simulink model "winter_simulink_with_PC_sim4"  (R2022a)
settings: Solver=VariableStepAuto  StartTime=0  StopTime=stop_time  FixedStep=simulation.time_step_H
undefined symbols (not defined in the file or in its folder): blade, Gc, gearbox, generator, I_eq, lambda_vector, lookup_cP, omega_R, omega_rated, pitch_range, pitch_vector, rho, Riq, rotor, simulation, wind, Yiq
settings Model: Creator=Niccolò  LastModifiedBy=Niccolò

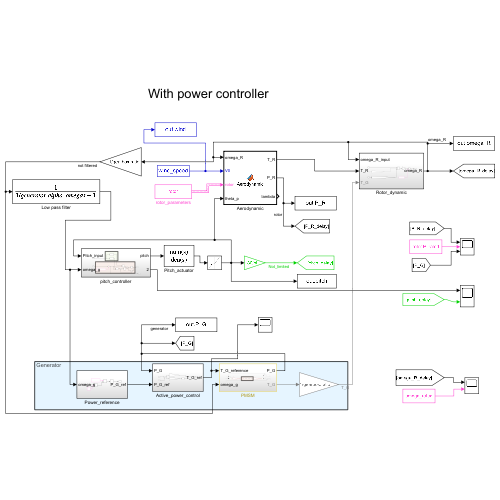
[thumbnail: Simulink's stored preview of the top-level diagram]
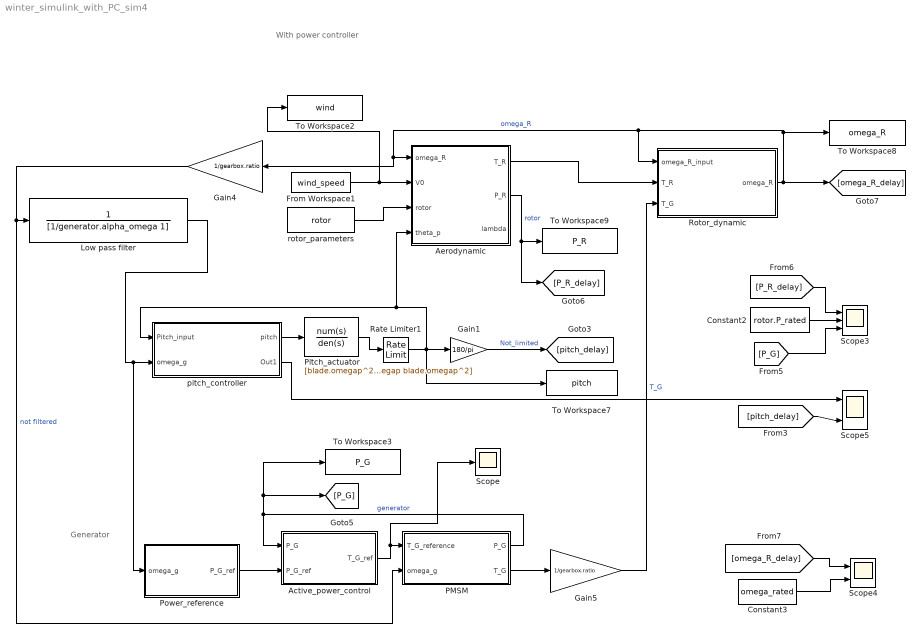
== system winter_simulink_with_PC_sim4 ==
  note: Generator
  note: With power controller
  Active_power_control : Subsystem
  Aerodynamic : MATLAB Function  TreatAsAtomicUnit=on
  Constant2 : Constant  Value=rotor.P_rated
  Constant3 : Constant  Value=omega_rated
  From Workspace1 : FromWorkspace  VariableName=wind_speed  SampleTime=1/wind.sample_f
  Gain1 : Gain  Gain=180/pi  SampleTime=simulation.time_step_H
  Gain4 : Gain  Gain=1/gearbox.ratio
  Gain5 : Gain  Gain=1/gearbox.ratio
  Low pass filter : TransferFcn  Denominator=[1/generator.alpha_omega 1]
  PMSM : Subsystem
  Pitch_actuator : TransferFcn  Numerator=[blade.omegap^2]  Denominator=[1 2*blade.zetap*blade.omegap blade.omegap^2]
  Power_reference : Subsystem
  Rate Limiter1 : RateLimiter  RisingSlewLimit=blade.pitch_rate  FallingSlewLimit=-blade.pitch_rate  SampleTimeMode=inherited
  Rotor_dynamic : Subsystem
  Scope : Scope
  Scope3 : Scope  NumInputPorts=3
  Scope4 : Scope  NumInputPorts=2
  Scope5 : Scope  NumInputPorts=2
  To Workspace2 : ToWorkspace  VariableName=wind  SaveFormat=Timeseries  SampleTime=-1
  To Workspace3 : ToWorkspace  VariableName=P_G  SaveFormat=Timeseries  SampleTime=-1
  To Workspace7 : ToWorkspace  VariableName=pitch  SaveFormat=Timeseries  SampleTime=-1
  To Workspace8 : ToWorkspace  VariableName=omega_R  SaveFormat=Timeseries  SampleTime=-1
  To Workspace9 : ToWorkspace  VariableName=P_R  SaveFormat=Timeseries  SampleTime=-1
  pitch_controller : Subsystem
  rotor_parameters : Constant  Value=rotor  OutDataTypeStr=Bus: rotor_bus
  wires:
  From Workspace1/1 -> To Workspace2/1, Aerodynamic/2(V0)
  Aerodynamic/2(P_R) -> [P_R_delay], To Workspace9/1  "rotor"
  [pitch_delay] -> Scope5/2
  Gain4/1 -> PMSM/2(omega_g), Low pass filter/1  "not filtered"
  Rate Limiter1/1 -> Aerodynamic/4(theta_p), pitch_controller/1(Pitch_input), Gain1/1, To Workspace7/1
  [P_R_delay] -> Scope3/1
  Constant3/1 -> Scope4/2
  Constant2/1 -> Scope3/2
  [omega_R_delay] -> Scope4/1
  Low pass filter/1 -> Power_reference/1(omega_g), pitch_controller/2(omega_g)
  Gain1/1 -> [pitch_delay]  "Not_limited"
  Gain5/1 -> Rotor_dynamic/3(T_G)  "T_G"
  PMSM/2(T_G) -> Gain5/1
  Aerodynamic/1(T_R) -> Rotor_dynamic/2(T_R)
  [P_G] -> Scope3/3
  rotor_parameters/1 -> Aerodynamic/3(rotor)
  PMSM/1(P_G) -> Active_power_control/1(P_G), To Workspace3/1, [P_G]  "generator"
  Power_reference/1(P_G_ref) -> Active_power_control/2(P_G_ref)
  Active_power_control/1(T_G_ref) -> Scope/1, PMSM/1(T_G_reference)
  Rotor_dynamic/1(omega_R) -> Gain4/1, Aerodynamic/1(omega_R), Rotor_dynamic/1(omega_R_input), To Workspace8/1, [omega_R_delay]  "omega_R"
  pitch_controller/1(pitch) -> Pitch_actuator/1
  pitch_controller/2(Out1) -> Scope5/1
  Pitch_actuator/1 -> Rate Limiter1/1

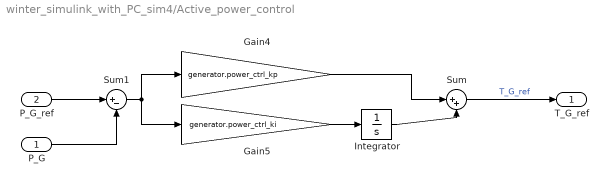
== system winter_simulink_with_PC_sim4/Active_power_control ==
  P_G : Inport
  P_G_ref : Inport  Port=2
  Gain4 : Gain  Gain=generator.power_ctrl_kp
  Gain5 : Gain  Gain=generator.power_ctrl_ki
  Integrator : Integrator
  Sum : Sum  Inputs=|++
  Sum1 : Sum  Inputs=|+-
  T_G_ref : Outport
  wires:
  P_G/1 -> Sum1/2
  Gain5/1 -> Integrator/1
  Sum1/1 -> Gain4/1, Gain5/1
  Sum/1 -> T_G_ref/1  "T_G_ref"
  Gain4/1 -> Sum/1
  Integrator/1 -> Sum/2
  P_G_ref/1 -> Sum1/1

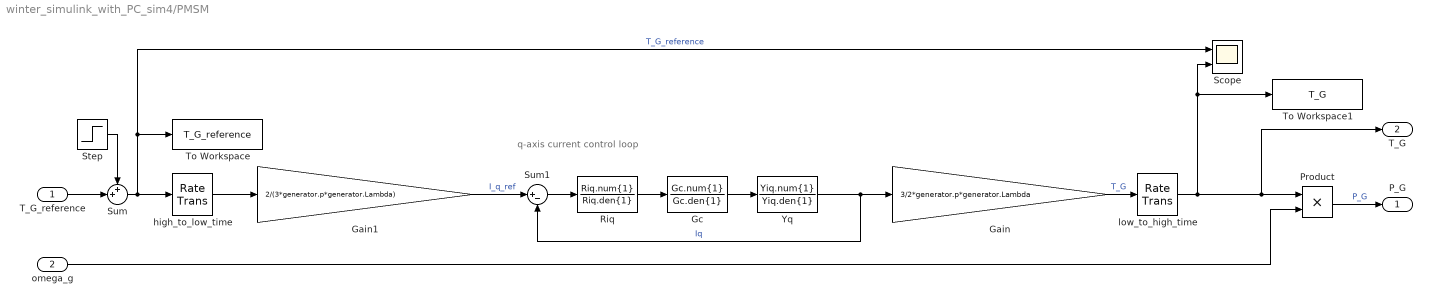
== system winter_simulink_with_PC_sim4/PMSM ==
  note: q-axis current control loop
  T_G_reference : Inport
  omega_g : Inport  Port=2
  Gain : Gain  Gain=3/2*generator.p*generator.Lambda  SampleTime=simulation.time_step_L
  Gain1 : Gain  Gain=2/(3*generator.p*generator.Lambda)  SampleTime=simulation.time_step_L
  Gc : TransferFcn  Numerator=Gc.num{1}  Denominator=Gc.den{1}
  Product : Product
  Riq : TransferFcn  Numerator=Riq.num{1}  Denominator=Riq.den{1}
  Scope : Scope  NumInputPorts=2
  Step : Step  Time=0.5  SampleTime=0
  Sum : Sum  Inputs=++|
  Sum1 : Sum  Inputs=|+-  SampleTime=simulation.time_step_L
  To Workspace : ToWorkspace  VariableName=T_G_reference  SaveFormat=Timeseries  SampleTime=-1
  To Workspace1 : ToWorkspace  VariableName=T_G  SaveFormat=Timeseries  SampleTime=-1
  Yq : TransferFcn  Numerator=Yiq.num{1}  Denominator=Yiq.den{1}
  high_to_low_time : RateTransition  OutPortSampleTime=simulation.time_step_L
  low_to_high_time : RateTransition
  P_G : Outport
  T_G : Outport  Port=2
  wires:
  Gc/1 -> Yq/1
  Gain/1 -> low_to_high_time/1  "T_G"
  Riq/1 -> Gc/1
  Sum1/1 -> Riq/1
  Yq/1 -> Gain/1, Sum1/2  "Iq"
  Product/1 -> P_G/1  "P_G"
  omega_g/1 -> Product/2
  Gain1/1 -> Sum1/1  "I_q_ref"
  high_to_low_time/1 -> Gain1/1
  low_to_high_time/1 -> T_G/1, Product/1, Scope/2, To Workspace1/1
  Sum/1 -> Scope/1, To Workspace/1, high_to_low_time/1  "T_G_reference"
  T_G_reference/1 -> Sum/2
  Step/1 -> Sum/1

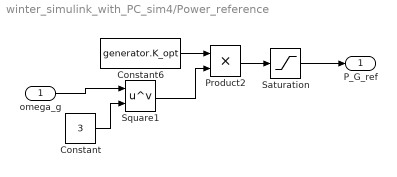
== system winter_simulink_with_PC_sim4/Power_reference ==
  omega_g : Inport
  Constant : Constant  Value=3
  Constant6 : Constant  Value=generator.K_opt
  Product2 : Product
  Saturation : Saturate  UpperLimit=rotor.P_rated  LowerLimit=0
  Square1 : Math  Operator=pow
  P_G_ref : Outport
  wires:
  Product2/1 -> Saturation/1
  omega_g/1 -> Square1/1
  Square1/1 -> Product2/2
  Constant6/1 -> Product2/1
  Saturation/1 -> P_G_ref/1
  Constant/1 -> Square1/2

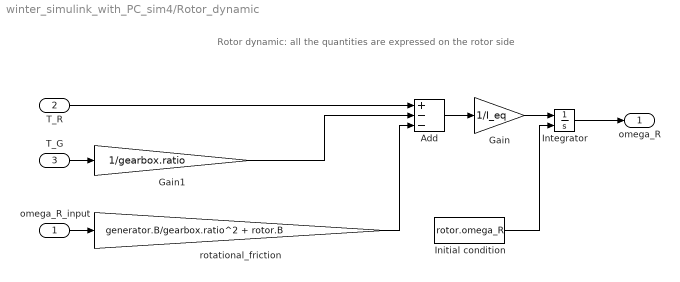
== system winter_simulink_with_PC_sim4/Rotor_dynamic ==
  note: Rotor dynamic: all the quantities are expressed on the rotor side
  omega_R_input : Inport
  T_R : Inport  Port=2
  T_G : Inport  Port=3
  Add : Sum  Inputs=+--
  Gain : Gain  Gain=1/I_eq
  Gain1 : Gain  Gain=1/gearbox.ratio
  Initial condition : Constant  Value=rotor.omega_R
  Integrator : Integrator  InitialConditionSource=external  InitialCondition=omega_R
  rotational_friction : Gain  Gain=generator.B/gearbox.ratio^2 + rotor.B
  omega_R : Outport
  wires:
  Add/1 -> Gain/1
  Gain/1 -> Integrator/1
  T_R/1 -> Add/1
  Initial condition/1 -> Integrator/2
  omega_R_input/1 -> rotational_friction/1
  rotational_friction/1 -> Add/3
  T_G/1 -> Gain1/1
  Gain1/1 -> Add/2
  Integrator/1 -> omega_R/1

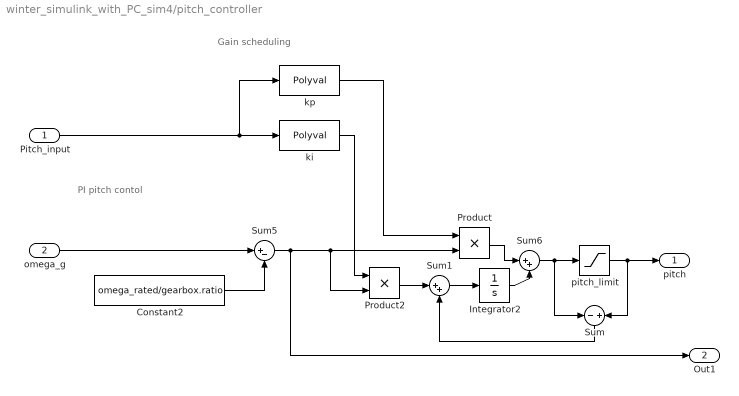
== system winter_simulink_with_PC_sim4/pitch_controller ==
  note: Gain scheduling
  note: PI pitch contol
  Pitch_input : Inport
  omega_g : Inport  Port=2
  Constant2 : Constant  Value=omega_rated/gearbox.ratio
  Integrator2 : Integrator
  Product : Product
  Product2 : Product
  Sum : Sum  Inputs=-|+
  Sum1 : Sum  Inputs=|++
  Sum5 : Sum  Inputs=|+-
  Sum6 : Sum  Inputs=|++
  ki : Polyval  Coefs=blade.ki_schedule
  kp : Polyval  Coefs=blade.kp_schedule
  pitch_limit : Saturate  UpperLimit=pitch_range(2)  LowerLimit=0
  pitch : Outport
  Out1 : Outport  Port=2
  wires:
  omega_g/1 -> Sum5/1
  Product/1 -> Sum6/1
  Constant2/1 -> Sum5/2
  ki/1 -> Product2/1
  kp/1 -> Product/1
  Pitch_input/1 -> kp/1, ki/1
  Sum6/1 -> Sum/1, pitch_limit/1
  Integrator2/1 -> Sum6/2
  pitch_limit/1 -> Sum/2, pitch/1
  Sum5/1 -> Product/2, Product2/2, Out1/1
  Sum1/1 -> Integrator2/1
  Product2/1 -> Sum1/1
  Sum/1 -> Sum1/2

== matlab function winter_simulink_with_PC_sim4/Aerodynamic ==
  data: omega_R input; V0 input; T_R output; P_R output; rho parameter; rotor input; theta_p input; lambda_vector parameter; pitch_vector parameter; lookup_cP parameter; lambda output
function [T_R, P_R, lambda] = Aerodynamic(omega_R, V0, rho, rotor, ...
  theta_p, lambda_vector, pitch_vector, lookup_cP) 

R = rotor.R;                  % rotor radius [m]

% retrive the cP from the look-up table
lambda = omega_R*R/V0;                                                
cP = interp2(lambda_vector, pitch_vector, lookup_cP, lambda, theta_p);

P_R = 0.5*rho*V0^3*pi*R^2*cP; % rotor power [W]
T_R = P_R/omega_R;            % rotor torque [Nm]
